simulink library "EmptyTranslation"  (R2022b)
settings: Solver=VariableStepAuto  StartTime=0.0  StopTime=10.0  RelTol=1e-3
settings Model: Creator=kl13806  LastModifiedBy=kl13806
settings SolverCC: AlgebraicLoopSolver=TrustRegion
settings DebuggingCC: UnconnectedInputMsg=warning  UnconnectedOutputMsg=warning  UnconnectedLineMsg=warning  SFMachineParentedDataDiag=warning  ArithmeticOperatorsInVariantConditions=warning
settings ModelReferenceCC: EnableRefExpFcnMdlSchedulingChecks=on
settings SFSimCC: SimUseLocalCustomCode=off  CustomCodeUndefinedFunction=UseInterfaceOnly
settings RTWCC: RTWUseLocalCustomCode=off  DLArmComputeVersion=19.05

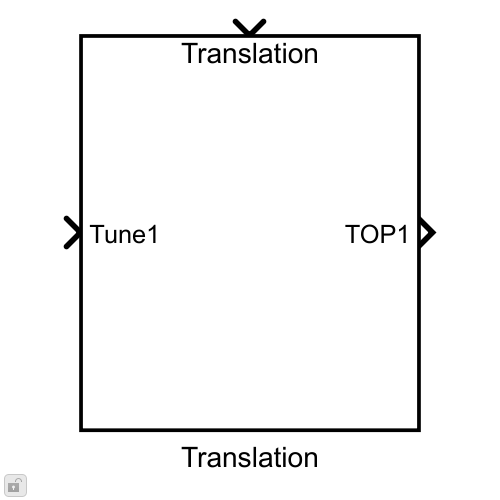
[thumbnail: Simulink's stored preview of the top-level diagram]
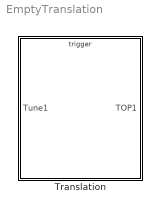
== system EmptyTranslation ==
  Translation : MATLAB Function  TreatAsAtomicUnit=on  mask(Talaria Translation){}
      mask help: This MATLAB Function Block can be automatically inserted by several automation routines. Once placed, the block is ready to accept translation logic from the model designer.

== matlab function EmptyTranslation/Translation ==
  data: TOP1 output; Tune1 input
  events: trigger input FUNCTION_CALL_EVENT
function TOP1  = fcn(Tune1)
%#codegen

% ----- To access TuneVar maximum size, current size, and current value:
%   Note: TuneVar signals arrive with exposed variable size information.
%         The expressions below illustrate for the "Tune1" input argument.
%
%   size(Tune1.Value) : the maximum possible size of the Tune1 variable
%
%   Tune.Size   : the current size of *valid* data in Tune1.Value
%
%   Tune1.Size(x) : Number of elements in dimension "x" that are currently
%   being used & contain valid data now. This count can be less than the
%   corresponding number in the dimensions from size(Tune1.Value) when the
%   TuneVar has specified that its variable dimension is dimension "x".
%   See "Variable Sizes" in https://wiki.bose.com/x/T5LoB
%
%   Tune1.Value : the current value of the tune variable... but end-padded 
%       to the maximum available size with undefined/invalid data.
%
%   numel(Tune1.Value) : another way of looking at the maximum number of
%       elements that could arrive in Tune1.Value
%
% ----- To register an error, use the following method (works like printf):
%   TranslateError( <format string>, <arguments ... )
%   ... this error will cause the build process to abort.
% ----- For warnings (works like printf):
%   TranslateWarning( <format string>, <arguments ... )
%   ... this warning will not set the translation engine error state.
%
% Note that TranslateError and TranslateWarning only work for code destined
% for the translation engine! If the code below might sometimes run on the
% DSP target, then special syntax tricks must be used to differentiate when
% to use error vs. TranslateError (e.g. existence of an optional argument)

% A trivial pass-through translation looks like this:
TOP1 = Tune1.Value;
